simulink model "full_bridge_new (1)"  (R2021a)
settings: Solver=VariableStepAuto  StartTime=0.0  StopTime=10  RelTol=1e-3
InitFcn:
  | fsw=20000
  | ts=1/fsw
libraries: spsIGBTDiodeLib x4, spsCurrentMeasurementLib x3, spsSeriesRLCBranchLib x3, spsDiodeLib x2, simulink x2, spsVoltageMeasurementLib x2, spsDCVoltageSourceLib x1, spsMultiWindingTransformerLib x1, spspowerguiLib x1
settings Model: OrderedModelArguments=off  Creator=Rohan  LastModifiedBy=Rohan
settings SolverCC: ZeroCrossAlgorithm=Adaptive
settings DebuggingCC: IgnoredZcDiagnostic=none

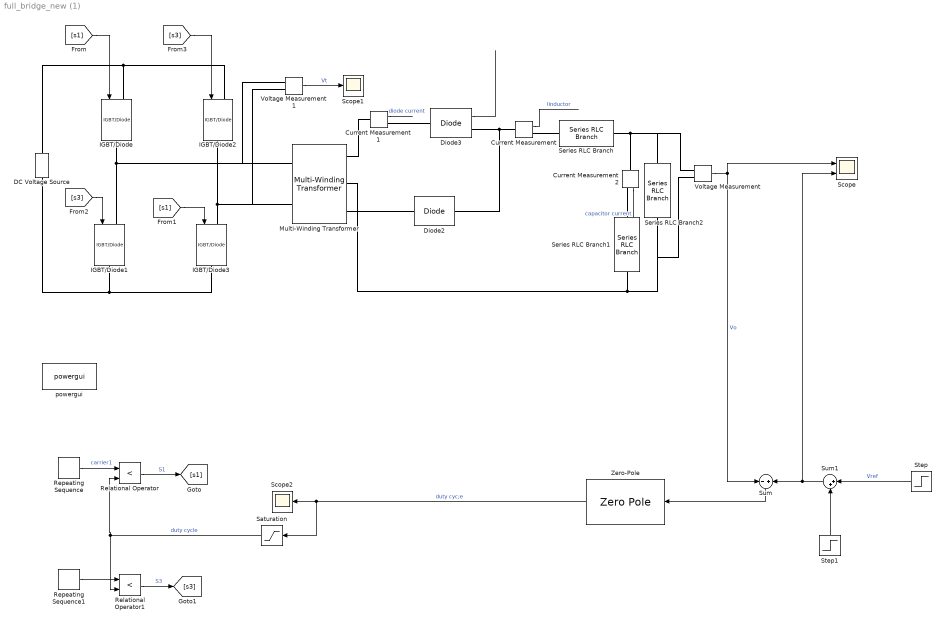
== system full_bridge_new (1) ==
  Current Measurement : spsCurrentMeasurementLib/Current Measurement  PhasorSimulation=off  OutputType=Complex  PSBequivalent=0
  Current Measurement1 : spsCurrentMeasurementLib/Current Measurement  PhasorSimulation=off  OutputType=Complex  PSBequivalent=0
  Current Measurement2 : spsCurrentMeasurementLib/Current Measurement  PhasorSimulation=off  OutputType=Complex  PSBequivalent=0
  DC Voltage Source : spsDCVoltageSourceLib/DC Voltage Source  Amplitude=400  Measurements=None
  Diode2 : spsDiodeLib/Diode  Ron=1e-8  Lon=0  Vf=0  IC=0  UseSnubber=0  Rs=0.0005  Cs=40e-9  Measurements=off
  Diode3 : spsDiodeLib/Diode  Ron=1e-8  Lon=0  Vf=0.0  IC=0  UseSnubber=0  Rs=0.0005  Cs=40e-9  Measurements=on
  IGBT/Diode{,1..3} (4 alike) : spsIGBTDiodeLib/IGBT//Diode  Ron=1e-3  Rs=1e5  Cs=inf  Measurements=off
  Multi-Winding Transformer : spsMultiWindingTransformerLib/Multi-Winding Transformer  LeftWindings=1  RightWindings=1  TappedWindings=taps on upper right winding  NumberOfTaps=1  SetSaturation=off  Hysteresis=off  DataFile='hysteresis.mat'  Measurements=None  UNITS=SI  NominalPower=[75e3 20000]  NominalVoltages=[ 400 400]  WindingResistances=[0 0]  WindingInductances=[0 0]  Rm=Inf  Lm=0.00125  Saturation=[0 0;168.75 2.4317e-05;70314 3.0802e-05]  BreakLoop=off  DiscreteSolver=Trapezoidal iterative  DataType=on  InitialFlux=0  TransfoNumber=1
      settings: SourceProductBaseCode=PS
  Relational Operator : RelationalOperator  Operator=<  OutDataTypeStr=boolean  RndMeth=Simplest
  Relational Operator1 : RelationalOperator  Operator=<  OutDataTypeStr=boolean  RndMeth=Simplest
  Repeating Sequence : simulink/Sources/Repeating Sequence  rep_seq_t=[0 1/8 2/8 3/8 4/8 5/8 6/8 7/8 8/8]*ts  rep_seq_y=[0.5 0 0.5 1 1.5 2 1.5 1 0.5]
  Repeating Sequence1 : simulink/Sources/Repeating Sequence  rep_seq_t=[0 1/8 2/8 3/8 4/8 5/8 6/8 7/8 8/8]*ts  rep_seq_y=[1.5 2 1.5 1 0.5 0 0.5 1 1.5]
  Saturation : Saturate  UpperLimit=1  LowerLimit=0  ZeroCross=off
  Scope : Scope  NumInputPorts=2
  Scope1 : Scope
  Scope2 : Scope
  Series RLC Branch : spsSeriesRLCBranchLib/Series RLC Branch  LConnTagsString=__new0  RConnTagsString=__new0  BranchType=L  Resistance=1  Inductance=218.9e-6  SetiL0=off  InitialCurrent=0  Capacitance=1e-6  Setx0=off  InitialVoltage=0  Measurements=None
  Series RLC Branch1 : spsSeriesRLCBranchLib/Series RLC Branch  LConnTagsString=__new0  RConnTagsString=__new0  BranchType=C  Resistance=1  Inductance=1e-3  SetiL0=off  InitialCurrent=0  Capacitance=6.78e-6  Setx0=off  InitialVoltage=0  Measurements=None
  Series RLC Branch2 : spsSeriesRLCBranchLib/Series RLC Branch  LConnTagsString=__new0  RConnTagsString=__new0  BranchType=R  Resistance=2.304  Inductance=1e-3  SetiL0=off  InitialCurrent=0  Capacitance=13.56e-6  Setx0=off  InitialVoltage=0  Measurements=None
  Step : Step  Time=0  After=48  SampleTime=0
  Step1 : Step  Time=2  After=30  SampleTime=0
  Sum : Sum  Inputs=-+
  Sum1 : Sum  Inputs=|++
  Voltage Measurement : spsVoltageMeasurementLib/Voltage Measurement  PhasorSimulation=off  OutputType=Complex  PSBequivalent=0
  Voltage Measurement1 : spsVoltageMeasurementLib/Voltage Measurement  PhasorSimulation=off  OutputType=Complex  PSBequivalent=0
  Zero-Pole : ZeroPole  Zeros=[-8000]  Poles=[ -0.08]  Gain=50e-5
  powergui : spspowerguiLib/powergui  Priority=1  SimulationMode=Discrete  SampleTime=1e-6  frequency=60  Iterations=50  frequencyindice=0  Pbase=100e6  ErrMax=1e-4  UnitsV=kV  UnitsW=MW  buscounter=0  FunctionMessages=off  echomessages=off  EnableUseOfTLC=off  CurrentSourceSwitches=off  DisableSnubberDevices=off  DisableRonSwitches=off  DisableVfSwitches=off  DisplayEquations=off  AutomaticDiscreteSolvers=off  SolverType=Tustin/Backward Euler (TBE)  Interpol=off  ExternalGateDelay=off  methode=off  Ts=100  x0status=blocks  SPID=on  SwTol=0  HookPort=off  NonlinearTolerance=1e-4  nMaxIteration=100  ContinueOnMaxIteration=off  RestoreLinks=warning  ResistiveCurrentMeasurement=off  Frange=[0:2:500]  Ylog=off  Xlog=on  ShowGrid=off  save=off  variable=ZData  structure=0  ZoomFFT=off  StartTime=0.0  cycles=1  DisplayStyle=1  fundamental=60  FreqAxis=off  MaxFrequency=1000  frequencyindicesteady=1  RmsSteady=1  display=off
  wires:
  [s1] -> IGBT/Diode/1
  [s1] -> IGBT/Diode3/1
  [s3] -> IGBT/Diode2/1
  Voltage Measurement/1 -> Scope/1, Sum/1  "Vo"
  Voltage Measurement1/1 -> Scope1/1  "Vt"
  Step/1 -> Sum1/1  "Vref"
  Sum1/1 -> Sum/2, Scope/2
  Current Measurement/1 -> ?  "Iinductor"
  Step1/1 -> Sum1/2
  [s3] -> IGBT/Diode1/1
  Relational Operator/1 -> [s1]  "S1"
  Relational Operator1/1 -> [s3]  "S3"
  Repeating Sequence1/1 -> Relational Operator1/1
  Repeating Sequence/1 -> Relational Operator/1  "carrier1"
  Sum/1 -> Zero-Pole/1
  Current Measurement1/1 -> ?  "diode current"
  Diode3/1 -> ?
  Current Measurement2/1 -> ?  "capacitor current"
  Saturation/1 -> Relational Operator/2, Relational Operator1/2  "duty cycle"
  Zero-Pole/1 -> Saturation/1, Scope2/1  "duty cyc;e"
  connections:
  DC Voltage Source/RConn1 -- IGBT/Diode2/LConn1 -- IGBT/Diode/LConn1
  DC Voltage Source/LConn1 -- IGBT/Diode1/RConn1 -- IGBT/Diode3/RConn1
  IGBT/Diode1/LConn1 -- Multi-Winding Transformer/LConn1 -- Voltage Measurement1/LConn1 -- IGBT/Diode/RConn1
  IGBT/Diode2/RConn1 -- Multi-Winding Transformer/LConn2 -- Voltage Measurement1/LConn2 -- IGBT/Diode3/LConn1
  Series RLC Branch/RConn1 -- Voltage Measurement/LConn1 -- Series RLC Branch2/LConn1 -- Current Measurement2/LConn1
  Diode2/LConn1 -- Multi-Winding Transformer/RConn3
  Current Measurement1/LConn1 -- Multi-Winding Transformer/RConn1
  Multi-Winding Transformer/RConn2 -- Series RLC Branch2/RConn1 -- Voltage Measurement/LConn2 -- Series RLC Branch1/RConn1
  Diode2/RConn1 -- Diode3/RConn1 -- Current Measurement/LConn1
  Current Measurement/RConn1 -- Series RLC Branch/LConn1
  Diode3/LConn1 -- Current Measurement1/RConn1
  Current Measurement2/RConn1 -- Series RLC Branch1/LConn1
